simulink model "OMP"  (R2023b)
settings: Solver=VariableStepAuto  StartTime=0.0  StopTime=10  RelTol=1e-3
values from neighbouring files (symbols this model uses):
  openmanipulator_pro = SerialLink(L, 'name', 'OpenManipulator-Pro')    [OMPro.m]    (also in OMPro_v1.m)
  qn = [0, pi/4, pi, 0, pi/4, 0]    [OMPro.m]    (also in OMPro_v1.m = [0, -pi/4, 0, 0, pi/4, 0]; OManPro.m = rand(1,6); moron9dof.m = [0.1 0.1 pi/4 pi/4 -pi/4 pi/4 0 pi/4 0]; testing2.m = [0 pi/4 pi/4 0 pi/4 0])
undefined symbols (not defined in the file or in its folder): cinertia
libraries: roblocks x10, robotmobilelib x1
settings Model: Creator=kangwang  LastModifiedBy=kangwang

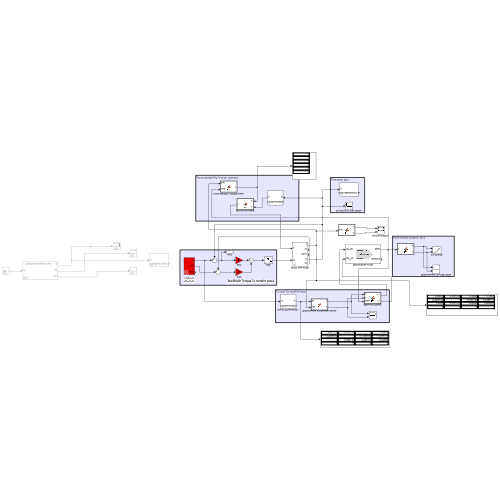
[thumbnail: Simulink's stored preview of the top-level diagram]
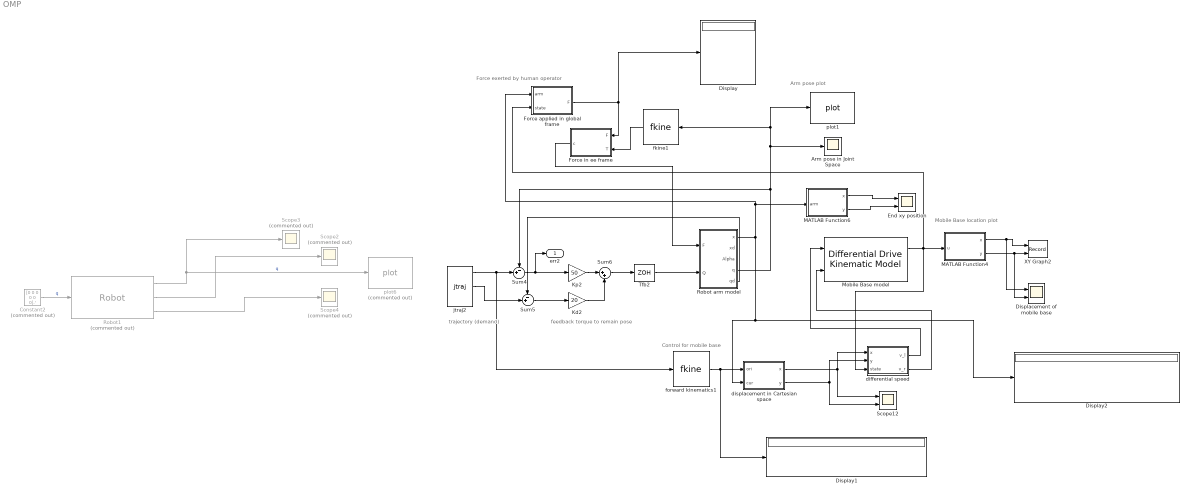
== system OMP ==
  note: trajectory
      | (demand)
  note: Mobile Base location plot
  note: Arm pose plot
  note: Control for mobile base
  note: Force exerted by human operator
  note: feedback torque to remain pose
  Arm pose in Joint Space : Scope
  Constant2 : Constant  Commented=on  Value=[0 0 0 0 0 0].'
  Displacement of mobile base : Scope  NumInputPorts=2
  Display : Display
  Display1 : Display
  Display2 : Display
  End xy position : Scope  NumInputPorts=2
  Force applied in global frame : MATLAB Function  TreatAsAtomicUnit=on
  Force in ee frame : MATLAB Function  TreatAsAtomicUnit=on
  Kd2 : Gain  Gain=20  SaturateOnIntegerOverflow=on  OutDataTypeStr=Inherit: Same as input  ParamDataTypeStr=Inherit: Same as input
  Kp2 : Gain  Gain=50  SaturateOnIntegerOverflow=on  OutDataTypeStr=Inherit: Same as input  ParamDataTypeStr=Inherit: Same as input
  MATLAB Function4 : MATLAB Function  TreatAsAtomicUnit=on
  MATLAB Function6 : MATLAB Function  TreatAsAtomicUnit=on
  Mobile Base model : robotmobilelib/Differential Drive Kinematic Model  VehicleInputs=Wheel Speeds  WheelRadius=0.05  WheelSpeedRange=[-inf inf]  TrackWidth=0.2  InitialState=[0; 0; 0]  SimulateUsing=Interpreted execution
  Robot arm model : Subsystem  mask{robot=openmanipulator_pro.nofriction, q0=qn}
      mask prompts: q0 "Initial joint angles"
  Robot1 : roblocks/Arm/Robot  Commented=on  robot=openmanipulator_pro.nofriction  q0=[0 0 0 0 0 0]
      link override Integrator1: InitialCondition=[0 0 0 0 0 0]
  Scope12 : Scope  NumInputPorts=2
  Scope2 : Scope  Commented=on
  Scope3 : Scope  Commented=on
  Scope4 : Scope  Commented=on
  Sum4 : Sum  Inputs=-+|  InputSameDT=on  SaturateOnIntegerOverflow=on  OutDataTypeStr=Inherit: Same as first input
  Sum5 : Sum  Inputs=-+|  InputSameDT=on  SaturateOnIntegerOverflow=on  OutDataTypeStr=Inherit: Same as first input
  Sum6 : Sum  Inputs=|++  InputSameDT=on  SaturateOnIntegerOverflow=on  OutDataTypeStr=Inherit: Same as first input
  Tfb2 : ZeroOrderHold  SampleTime=0.002
  XY Graph2 : Record  FileSettingsInternal="{\"entries\":[{\"content\":{\"excelSettings\":{\"content\":{},\"type\":\"Streamout.ExcelSettings\"}},\"type\":\"Streamout.FileSettingStorage\",\"uuid\":\"\"}],\"packageUris\":[\"http:\\/\\/schema.mathworks.com\\/mf0\\/streamout_blocks\\/R2020a\"],\"version\":\"1.0\"}"  Layout=[1 1]  SignalsInternal="{\"entries\":[{\"content\":{\"signals\":[{\"content\":{\"blockPath\":[],\"dimensions\":[1],\"domain\":\"\",\"lineColor\":\"#64d413\",\"plots\":[1],\"port\":1,\"sid\":[\"\"],\"signalID\":24,\"signalName\":\"MATLAB Function4:1\"},\"type\":\"RecordBlkView.Signal\",\"uuid\":\"\"},{\"content\":{\"blockPath\":[],\"dimensions\":[1],\"domain\":\"\",\"lineColor\":\"#ff13a6\",\"plots\":[1],\"port\":2,\"sid\":[\"\"],\"signalID\":28,\"signalName\":\"MATLAB Function4:2\"},\"type\":\"RecordBlkView.Signal\",\"uuid\":\"\"}]},\"type\":\"RecordBlkView.InputSignals\",\"uuid\":\"\"}],\"packageUris\":[\"http:\\/\\/schema.mathworks.com\\/mf0\\/streamout_blocks\\/R2020a\"],\"version\":\"1.0\"}"  VisualizationBindings="{\"xyplotplugin\":{\"info\":[{\"series\":[{\"bindingParametersList\":[{\"parameter\":\"X-Axis\",\"signalID\":24,\"signalName\":\"MATLAB Function4:1\"},{\"parameter\":\"Y-Axis\",\"signalID\":28,\"signalName\":\"MATLAB Function4:2\"}],\"seriesID\":51558}],\"subplotID\":1}]}}"  CompatibilityTag=XY
  differential speed : MATLAB Function  TreatAsAtomicUnit=on
  displacement in Cartesian space : MATLAB Function  TreatAsAtomicUnit=on
  fkine1 : roblocks/Arm/fkine  robot=openmanipulator_pro.nofriction
  forward kinematics1 : roblocks/Arm/fkine  robot=openmanipulator_pro.nofriction
  jtraj2 : roblocks/Toolbox/jtraj  q0=qn  qf=qn  tmax=5  ts=0.02
  plot1 : roblocks/Arm/plot  robot=openmanipulator_pro.nofriction  fps=10  holdplot=on
  plot6 : roblocks/Arm/plot  Commented=on  robot=openmanipulator_pro.nofriction  fps=10  holdplot=on
  err2 : Outport
  wires:
  Robot1/3 -> Scope4/1
  Robot1/2 -> Scope2/1
  Constant2/1 -> Robot1/1  "q"
  Robot1/1 -> Scope3/1, plot6/1  "q"
  Force in ee frame/1(c) -> Robot arm model/1(F)
  Tfb2/1 -> Robot arm model/2(Q)
  Robot arm model/1(x) -> MATLAB Function6/1(arm), Force applied in global frame/1(arm), displacement in Cartesian space/2(cur), Display2/1
  Mobile Base model/1 -> differential speed/3(state), MATLAB Function4/1(u), Force applied in global frame/2(state)
  Sum6/1 -> Tfb2/1
  Robot arm model/4(q) -> plot1/1, fkine1/1, Arm pose in Joint Space/1, Sum4/1
  jtraj2/2 -> Sum5/2
  differential speed/2(v_r) -> Mobile Base model/2
  jtraj2/1 -> forward kinematics1/1, Sum4/2
  displacement in Cartesian space/1(x) -> differential speed/1(x), Scope12/1
  fkine1/1 -> Force in ee frame/2(T)
  MATLAB Function6/1(x) -> End xy position/1
  Robot arm model/5(qd) -> Sum5/1
  Sum4/1 -> err2/1, Kp2/1
  differential speed/1(v_l) -> Mobile Base model/1
  Kp2/1 -> Sum6/1
  MATLAB Function6/2(y) -> End xy position/2
  Force applied in global frame/1(F) -> Display/1, Force in ee frame/1(F)
  displacement in Cartesian space/2(y) -> differential speed/2(y), Scope12/2
  Sum5/1 -> Kd2/1
  Kd2/1 -> Sum6/2
  MATLAB Function4/1(x) -> Displacement of mobile base/1, XY Graph2/1
  MATLAB Function4/2(y) -> Displacement of mobile base/2, XY Graph2/2
  forward kinematics1/1 -> displacement in Cartesian space/1(ori), Display1/1

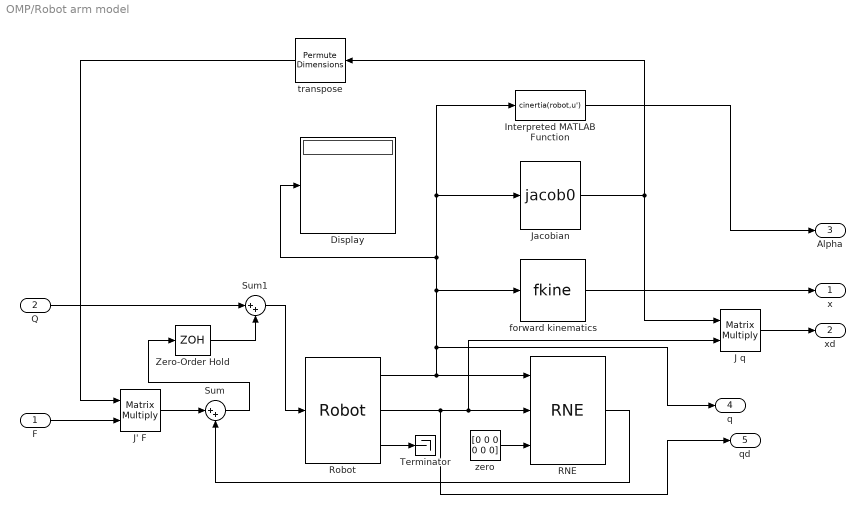
== system OMP/Robot arm model ==
  F : Inport
  Q : Inport  Port=2
  Display : Display
  Interpreted MATLAB Function : MATLABFcn  MATLABFcn=cinertia(robot,u')  OutputDimensions=[6 6]  Output1D=off
  J q : Product  Multiplication=Matrix(*)
  J' F : Product  Multiplication=Matrix(*)
  Jacobian : roblocks/Arm/jacob0   robot=robot
  RNE : roblocks/Arm/RNE  robot=robot  grav=[0 0 9.81]
  Robot : roblocks/Arm/Robot  robot=robot  q0=q0
  Sum : Sum  Inputs=|++
  Sum1 : Sum  Inputs=|++
  Terminator : Terminator
  Zero-Order Hold : ZeroOrderHold  SampleTime=5e-3
  forward kinematics : roblocks/Arm/fkine  robot=robot
  transpose : PermuteDimensions
  zero : Constant  Value=[0 0 0 0 0 0]
  x : Outport
  xd : Outport  Port=2
  Alpha : Outport  Port=3
  q : Outport  Port=4
  qd : Outport  Port=5
  wires:
  Interpreted MATLAB Function/1 -> Alpha/1
  Sum/1 -> Zero-Order Hold/1
  F/1 -> J' F/2
  transpose/1 -> J' F/1
  J' F/1 -> Sum/1
  zero/1 -> RNE/3
  Robot/3 -> Terminator/1
  Robot/2 -> qd/1, RNE/2, J q/2
  Robot/1 -> RNE/1, forward kinematics/1, Interpreted MATLAB Function/1, Jacobian/1, Display/1, q/1
  forward kinematics/1 -> x/1
  J q/1 -> xd/1
  Jacobian/1 -> transpose/1, J q/1
  Q/1 -> Sum1/1
  Sum1/1 -> Robot/1
  Zero-Order Hold/1 -> Sum1/2
  RNE/1 -> Sum/2

== matlab function OMP/Force in ee frame ==
  data: F input; T input; c output
function c = fcn(F, T)
y = inv(T(1:3,1:3))*F(1:3);
c = [y.', 0,0,0].';

== matlab function OMP/MATLAB Function4 ==
  data: x output; u input; y output
function [x,y]= fcn(u)

x = u(1);
y = u(2);

== matlab function OMP/displacement in Cartesian space ==
  data: x output; ori input; y output; cur input
function [x,y]= fcn(ori, cur)
x = cur(1,4)-ori(1,4);
y = cur(2,4)-ori(2,4);

== matlab function OMP/Force applied in global frame ==
  data: arm input; F output; state input
function F = fcn(arm,state)
x_arm = arm(1,4);
x_base = state(1);
y_arm = arm(2,4);
y_base = state(2);
x = x_base+x_arm;
y = y_base+y_arm;
F = [0 0 0 0 0 0].';
if x < 1.2 || y < 1.8 
    F = [5 0 0 0 0 0].';
end

== matlab function OMP/differential speed ==
  data: x input; y input; v_l output; v_r output; state input
function [v_l, v_r]= fcn(x, y, state)
    current_heading = state(3);           
    k_theta = 2.0;                    

    r = 0.05;                         
    L = 0.2;                          

    % Rebalancing y-direction influence
    y_scale = 0.522;  % Try values < 1 to reduce y influence
    x_scale = 1.0;  % Keep x unchanged (or tweak as needed)

    x_scaled = x_scale * x;
    y_scaled = y_scale * y;

    force_angle = atan2(y_scaled, x_scaled);

    % gain for the speed (also using scaled values)
    speed = 20 * norm([x_scaled, y_scaled]);

    error_theta = wrapToPi(force_angle - current_heading);
    w = k_theta * error_theta;

    v = speed;  

    v_l = (2*v - w*L)/(2*r);
    v_r = (2*v + w*L)/(2*r);
end

== matlab function OMP/MATLAB Function6 ==
  data: x output; arm input; y output
function [x,y]= fcn(arm)
x = arm(1,4);
y = arm(2,4);
